simulink model "EmulationDesign"  (R2024b)
settings: Solver=VariableStepAuto  StartTime=0.0  StopTime=10.0  RelTol=1e-3
values from neighbouring files (symbols this model uses):
  A = [0 1; -1 -2]    [ex1.m]
  B = [0; 1]    [ex1.m]
  C = [1 0]    [ex1.m]
  Cd = Gd_zoh    [ex1.m]
  D = 0    [ex1.m]
undefined symbols (not defined in the file or in its folder): dspblkCoreblockFVToolHelper, gcbh
settings Model: Creator=froessil  LastModifiedBy=froessil

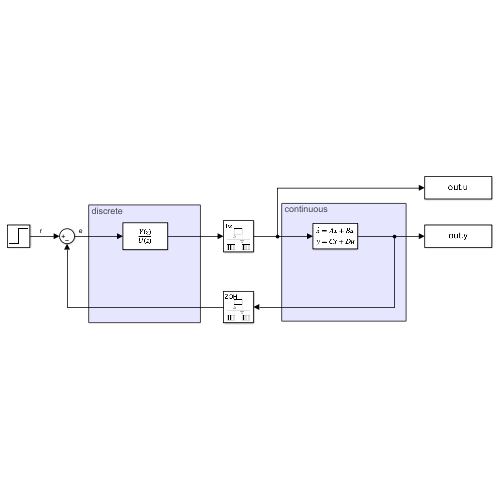
[thumbnail: Simulink's stored preview of the top-level diagram]
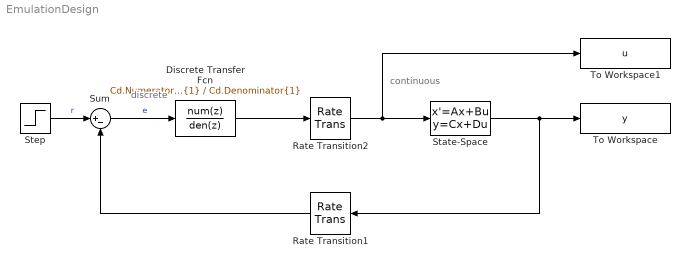
== system EmulationDesign ==
  note: discrete
  note: continuous
  Discrete Transfer Fcn : DiscreteTransferFcn  LoadFcn=dspblkCoreblockFVToolHelper(gcbh,'load');  Numerator=Cd.Numerator{1}  Denominator=Cd.Denominator{1}
      settings: CopyFcn=dspblkCoreblockFVToolHelper(gcbh,'copy');  DeleteFcn=dspblkCoreblockFVToolHelper(gcbh,'close');  ModelCloseFcn=dspblkCoreblockFVToolHelper(gcbh,'close');  PreSaveFcn=dspblkCoreblockFVToolHelper(gcbh,'presave');  PostSaveFcn=dspblkCoreblockFVToolHelper(gcbh,'postsave');  CloseFcn=dspblkCoreblockFVToolHelper(gcbh,'close');
  Rate Transition1 : RateTransition  OutPortSampleTime=T
  Rate Transition2 : RateTransition  OutPortSampleTime=0
  State-Space : StateSpace  A=A  B=B  C=C  D=D  InitialCondition=0
  Step : Step  Time=0  SampleTime=0
  Sum : Sum  Inputs=|+-
  To Workspace : ToWorkspace  VariableName=y  SaveFormat=Timeseries  SampleTime=-1
  To Workspace1 : ToWorkspace  VariableName=u  SaveFormat=Timeseries  SampleTime=-1
  wires:
  State-Space/1 -> Rate Transition1/1, To Workspace/1
  Rate Transition2/1 -> State-Space/1, To Workspace1/1
  Discrete Transfer Fcn/1 -> Rate Transition2/1
  Step/1 -> Sum/1  "r"
  Sum/1 -> Discrete Transfer Fcn/1  "e"
  Rate Transition1/1 -> Sum/2
